simulink model "s2dot2_bus_selector"  (R2023b)
settings: Solver=VariableStepAuto  StartTime=0.0  StopTime=10.0  RelTol=1e-3
settings Model: Creator=lxj  LastModifiedBy=lxj

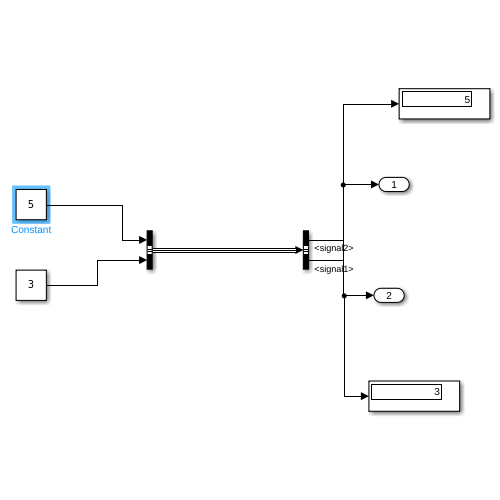
[thumbnail: Simulink's stored preview of the top-level diagram]
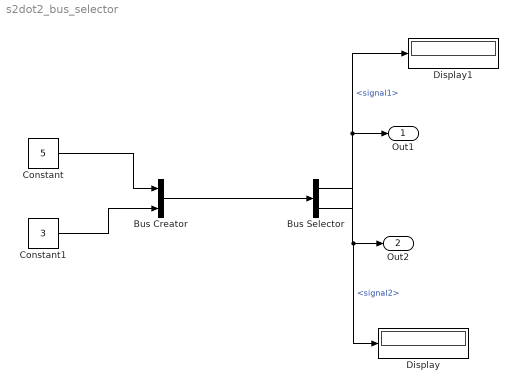
== system s2dot2_bus_selector ==
  Bus Creator : BusCreator  Inputs=2
  Bus Selector : BusSelector  OutputSignals=signal2,signal1
  Constant : Constant  Value=5
  Constant1 : Constant  Value=3
  Display : Display
  Display1 : Display
  Out1 : Outport
  Out2 : Outport  Port=2
  wires:
  Constant1/1 -> Bus Creator/2
  Constant/1 -> Bus Creator/1
  Bus Creator/1 -> Bus Selector/1
  Bus Selector/1 -> Display/1, Out2/1  "<signal2>"
  Bus Selector/2 -> Display1/1, Out1/1  "<signal1>"
